simulink model "power_wt_fuzzy"  (R2020a)
settings: Solver=VariableStepAuto  StartTime=0.0  StopTime=10.0  RelTol=1e-3
libraries: simulink x2, fuzblock x1
settings Model: Creator=asus  LastModifiedBy=asus

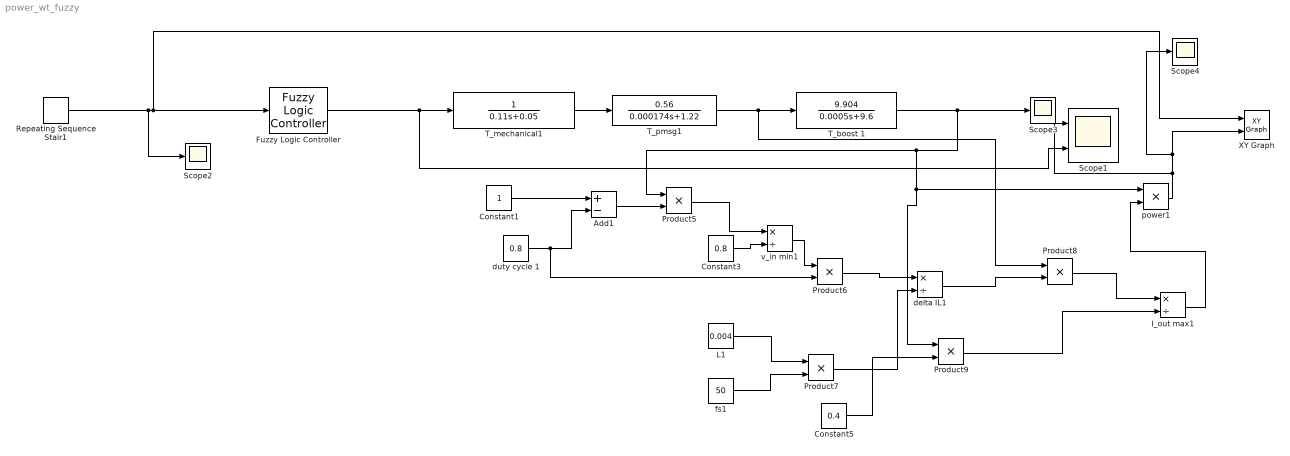
== system power_wt_fuzzy ==
  Add1 : Sum  Inputs=+-
  Constant1 : Constant
  Constant3 : Constant  Value=0.8
  Constant5 : Constant  Value=0.4
  Fuzzy Logic Controller : fuzblock/Fuzzy Logic  Controller  FIS=mppt  OutputSampleNumber=101  DataType=double  FuzzifiedInputs=off  RuleFiringStrengths=off  RuleOutputs=off  AggregatedOutputs=off  SimulateUsing=Interpreted execution  OutOfRangeInputValueMessage=warning  NoRuleFiredMessage=warning  EmptyOutputFuzzySetMessage=warning
  I_out max1 : Product  Inputs=*/
  L1 : Constant  Value=0.004
  Product{5..9} (5 alike) : Product
  Repeating Sequence Stair1 : simulink/Sources/Repeating Sequence Stair  OutValues=[4.5 5.1 6.2 6.6 7.1 4.2 8.3 9.1 8.2 7.7 9.9 9.8 8.9 7.6 6.2 6.4 6.8 6.9 4.2 5.1 5.2 6.3 5.8 7.2 4.4 8.2 9.1 8.8 4.8 5.2 6.8 6.9 6.3 5.4 5.5 5.8 10 6.2 6.4 8.8 9.2 7.3 9.2 8.5 8.9 7.7 7.8 7.9 4 5.1 4.2 4.3 5.6 5.6 5.6 9.1 7.8 6.9 5.2]  tsamp=-1  OutMin=[]  OutMax=[]  OutDataTypeStr=double  OutputDataTypeScalingMode=double  OutDataType=fixdt(0,8)  ConRadixGroup=Best Precision: Vector-wise  OutScaling=2^-12
  Scope1 : Scope  NumInputPorts=2
  Scope2 : Scope
  Scope3 : Scope
  Scope4 : Scope
  T_boost 1 : TransferFcn  Numerator=[9.904]  Denominator=[0.0005 9.6]
  T_mechanical1 : TransferFcn  Denominator=[0.11 0.05]
  T_pmsg1 : TransferFcn  Numerator=[0.56]  Denominator=[0.000174 1.22]
  XY Graph : simulink/Sinks/XY Graph  xmin=4  xmax=12  ymin=2876000  ymax=27340000  st=0
  delta IL1 : Product  Inputs=*/
  duty cycle 1 : Constant  Value=0.8
  fs1 : Constant  Value=50
  power1 : Product
  v_in min1 : Product  Inputs=*/
  wires:
  Product6/1 -> delta IL1/1
  Repeating Sequence Stair1/1 -> Fuzzy Logic Controller/1, XY Graph/1, Scope2/1
  T_pmsg1/1 -> Product8/1, T_boost 1/1
  duty cycle 1/1 -> Product6/2, Add1/2
  I_out max1/1 -> power1/2
  Product7/1 -> delta IL1/2
  v_in min1/1 -> Product6/1
  Constant1/1 -> Add1/1
  Add1/1 -> Product5/2
  fs1/1 -> Product7/2
  Product5/1 -> v_in min1/1
  delta IL1/1 -> Product8/2
  T_mechanical1/1 -> T_pmsg1/1
  Constant3/1 -> v_in min1/2
  Fuzzy Logic Controller/1 -> Scope1/2, T_mechanical1/1
  power1/1 -> Scope4/1, XY Graph/2, Scope1/1
  Constant5/1 -> Product9/2
  L1/1 -> Product7/1
  T_boost 1/1 -> Scope3/1, power1/1, Product9/1, Product5/1
  Product8/1 -> I_out max1/1
  Product9/1 -> I_out max1/2
